simulink model "cw4_zad12"  (R2020b)
settings: Solver=VariableStepAuto  StartTime=0.0  StopTime=10.0  RelTol=1e-3
undefined symbols (not defined in the file or in its folder): K_d_den, K_d_num, K_d_st, K_den, K_num
settings Model: Creator=johnb  LastModifiedBy=john

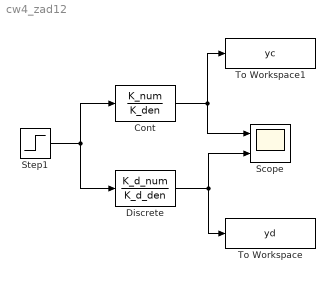
== system cw4_zad12 ==
  Cont : TransferFcn  Numerator=K_num  Denominator=K_den
  Discrete : DiscreteTransferFcn  Numerator=K_d_num  Denominator=K_d_den  SampleTime=K_d_st
  Scope : Scope  NumInputPorts=2
  Step1 : Step  SampleTime=0
  To Workspace : ToWorkspace  VariableName=yd  SaveFormat=Timeseries  SampleTime=K_d_st
  To Workspace1 : ToWorkspace  VariableName=yc  SaveFormat=Timeseries  SampleTime=-1
  wires:
  Step1/1 -> Discrete/1, Cont/1
  Cont/1 -> Scope/1, To Workspace1/1
  Discrete/1 -> To Workspace/1, Scope/2
